simulink model "position_signalGenerator"  (R2018b)
settings: Solver=FixedStepDiscrete  StartTime=0.0  StopTime=16  RelTol=1e-3
settings Model: ExtModeTrigDuration=2  Creator=sin29  LastModifiedBy=sin29
settings OptimizationCC: DefaultParameterBehavior=Inlined  UseDivisionForNetSlopeComputation=on  UseFloatMulNetSlope=on  InlineInvariantSignals=on  PassReuseOutputArgsAs=Individual arguments  ZeroExternalMemoryAtStartup=off  ZeroInternalMemoryAtStartup=off  NoFixptDivByZeroProtection=on  EfficientFloat2IntCast=on  LifeSpan=1  MaxStackSize=64  OptimizeBlockOrder=speed  DifferentSizesBufferReuse=on
settings DebuggingCC: ParameterTunabilityLossMsg=error
settings HardwareCC: ProdBitPerInt=16  ProdBitPerPointer=16  ProdBitPerSizeT=16  ProdBitPerPtrDiffT=16  ProdLargestAtomicFloat=None  ProdWordSize=8  ProdLongLongMode=on  ProdHWDeviceType=Atmel->AVR
settings SFSimCC: MATLABDynamicMemAlloc=off
settings RTWCC: SystemTargetFile=ert.tlc  HardwareBoard=Arduino Uno  TemplateMakefile=ert_default_tmf  GenerateReport=on  Toolchain=Arduino AVR  BuildConfiguration=Faster Runs  IncludeHyperlinkInReport=on  LaunchReport=on  GenerateTraceInfo=on  GenerateTraceReport=on  GenerateTraceReportSl=on  GenerateTraceReportSf=on  GenerateTraceReportEml=on  GenerateCodeMetricsReport=on
settings CodeAppCC: ForceParamTrailComments=on  IgnoreCustomStorageClasses=off  OperatorAnnotations=on  SimulinkDataObjDesc=on  SFDataObjDesc=on  CustomSymbolStrGlobalVar=rt$N$M  CustomSymbolStrType=$N$M  CustomSymbolStrFcn=$N$M$F  CustomSymbolStrMacro=$N$M  InsertBlockDesc=on
settings ERTTargetCC: IncludeMdlTerminateFcn=off  CombineSignalStateStructs=on  SupportComplex=off  SupportContinuousTime=on  SupportNonInlinedSFcns=on  InlinedParameterPlacement=NonHierarchical  ERTFilePackagingFormat=CompactWithDataFile  MemSecPackage=Simulink

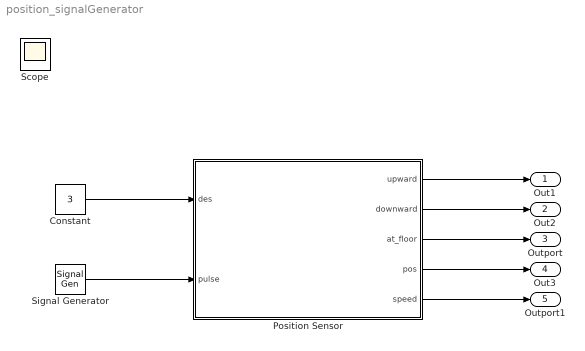
== system position_signalGenerator ==
  Constant : Constant  Value=3
  "Position Sensor " : Stateflow chart  TreatAsAtomicUnit=on
  Signal Generator : SignalGenerator  WaveForm=square  Frequency=50
  Out1 : Outport
  Out2 : Outport  Port=2
  Outport : Outport  Port=3
  Out3 : Outport  Port=4
  Outport1 : Outport  Port=5
  Scope : Scope
  wires:
  "Position Sensor "/1(upward) -> Out1/1
  "Position Sensor "/2(downward) -> Out2/1
  "Position Sensor "/3(at_floor) -> Outport/1
  Signal Generator/1 -> "Position Sensor "/2(pulse)
  Constant/1 -> "Position Sensor "/1(des)
  "Position Sensor "/4(pos) -> Out3/1
  "Position Sensor "/5(speed) -> Outport1/1

== stateflow chart position_signalGenerator/Position Sensor  ==
  state pos_detection
    state speed_cal [parallel]
      settings: executionOrder=1
      (history)
      state speed_at_1
        entry:
        speed = abs(pos - last_counter);
        last_counter = pos;
      (default) -> speed_at_1
      speed_at_1 -> speed_at_1 : [after(1,sec)]
    state pos_cal [parallel]
      settings: executionOrder=2
      (history)
      state floor_3
        entry:
        counter = 0;
        at_floor = 3;
        pos = 800;
        during:
        upward = 0;
        downward = 0;
      state floor_1
        entry:
        counter = 0;
        at_floor = 1;
        pos = 0;
        during:
        upward = 0;
        downward = 0;
      state between_1_2
        entry:
        at_floor = -1;
        pos = (upward)*(counter) + (downward)*(400 - counter)
        exit:
      state between_2_3
        entry:
        at_floor = -1;
        pos = (upward)*(counter+400) + (downward)*(800 - counter)
      state read_pulse_2_3
        entry:
        counter = counter+1
        last = pulse;
      state read_pulse_1_2
        entry:
        counter = counter+1
        last = pulse
      state floor_2
        entry:
        counter = 0;
        at_floor = 2;
        pos = 400;
        during:
        upward = 0;
        downward = 0;
      (default) -> floor_1
      read_pulse_2_3 -> floor_3 [order 1] : [counter == 400 && upward == 1]
      read_pulse_1_2 -> floor_1 [order 1] : [counter == 400 && downward == 1]
      floor_3 -> between_2_3 : [des == 2 || des == 1]{upward = 0 ; downward = 1}
      floor_1 -> between_1_2 : [des == 2 || des == 3]{upward = 1;downward = 0}
      between_1_2 -> between_1_2 [order 2] : [after(3,msec)&&last == pulse]
      read_pulse_1_2 -> between_1_2 [order 3] : [counter ~= 400]
      floor_2 -> between_2_3 [order 2] : [des == 3]{upward = 1; downward = 0}
      read_pulse_2_3 -> between_2_3 [order 3] : [counter ~= 400]
      between_2_3 -> read_pulse_2_3 : [after(3,msec)&& last ~= pulse]
      between_1_2 -> read_pulse_1_2 [order 1] : [after(3,msec)&& last ~= pulse]
      floor_2 -> between_1_2 [order 1] : [des == 1]{upward = 0;downward =1}
      read_pulse_2_3 -> floor_2 [order 2] : [counter == 400 && downward == 1]
      read_pulse_1_2 -> floor_2 [order 2] : [counter == 400 && upward == 1]
  state init
    exit :
    counter = 0;
    last_counter = 0;
    pos = 0;
  (default) -> init
  init -> pos_detection
  data: upward output; downward output; counter local; des input; last local; pulse input; at_floor output; pos output; speed output; last_counter local
